simulink model "motominiPlanning"  (R2019a)
settings: Solver=ode3  StartTime=0.0  StopTime=totalTime  FixedStep=1e-3  RelTol=1e-3
values from neighbouring files (symbols this model uses):
  MotominiParams = setMotominiParameters(ROS_master_ip,motomini)    [managePlannerRequests.m]
  obstacles = [colObject1]    [calcStartingTrajWithPlanner.m]    (also in managePlannerRequests.m = []; testTrajectoryPlanner.m = [])
  Qt = QOpt    [calcStartingTrajWithPlanner.m]    (also in planTrajectory.m; testTrajectoryPlanner.m)
  s = char(axisElement.getAttribute('xyz'))    [loadRobotFromURDF.m]    (also in testTrajectoryPlanner.m = patch(surf2patch(X,Y,Z)))
  X = X + cupPosition(1)    [testTrajectoryPlanner.m]
  Y = Y + cupPosition(2)    [testTrajectoryPlanner.m]
  Z = Z + cupPosition(3)    [testTrajectoryPlanner.m]
undefined symbols (not defined in the file or in its folder): X0, Xf
libraries: sm_lib x111, nesl_utility x70, sharedtransform x2, aerolibtransform2 x2, simulink x1
(part 1 of 4)
settings Model: Creator=tomvose  LastModifiedBy=tkikawad
settings DataIOCC: ReturnWorkspaceOutputs=off
settings DebuggingCC: PregeneratedLibrarySubsystemCodeDiagnostic=none  ArithmeticOperatorsInVariantConditions=warning
settings SFSimCC: SimUseLocalCustomCode=off
settings RTWCC: RTWUseLocalCustomCode=off
settings CodeAppCC: StateflowObjectComments=on
settings ConfigComp: CovMetricSettings=dswe
settings SimscapeCC: SimscapeNormalizeSystem=off
settings ExplorerConfigSet: SimMechanicsOpenEditorOnUpdate=off

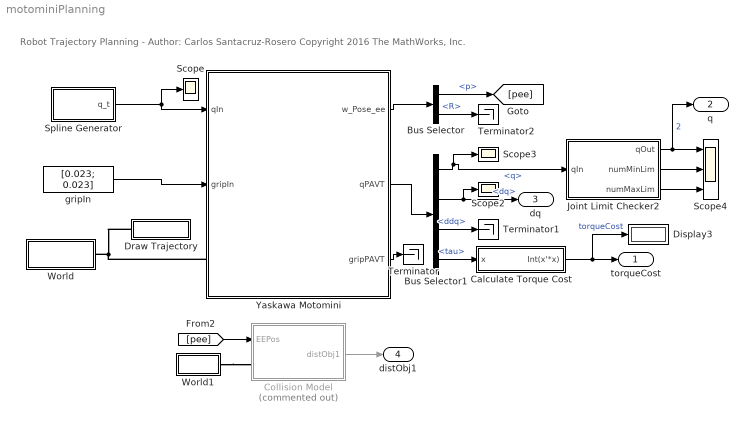
== system motominiPlanning ==
  note: Robot Trajectory Planning - Author: Carlos Santacruz-Rosero
      | Copyright 2016 The MathWorks, Inc.
  Bus Selector : BusSelector  OutputSignals=p,R
  Bus Selector1 : BusSelector  OutputSignals=q,dq,ddq,tau
  Calculate Torque Cost : Subsystem
  Collision Model : Subsystem  Commented=on
  Display3 : Display
  Draw Trajectory : Subsystem
  Joint Limit Checker2 : Subsystem  VariantControl="mode == OP2Model ||  mode == OP2ROS"
      mask Display:
      | plot([0.3 0.7], [0.5 0.5])
      | plot([0.3 0.4 0.6 0.7], [0.25 0.25 0.75 0.75])
  Scope : Scope
  Scope2 : Scope
  Scope3 : Scope
  Scope4 : Scope  NumInputPorts=3
  Spline Generator : Subsystem
  Terminator : Terminator
  Terminator1 : Terminator
  Terminator2 : Terminator
  World : Subsystem
  World1 : Subsystem
  Yaskawa Motomini : Subsystem
  gripIn : Constant  Value=[0.023; 0.023]
  torqueCost : Outport  SignalName=torqueCost
  q : Outport  Port=2  SignalName=q
  dq : Outport  Port=3  SignalName=dq
  distObj1 : Outport  Port=4  SignalName=distObj1
  wires:
  Spline Generator/1(q_t) -> Yaskawa Motomini/1(qIn), Scope/1
  gripIn/1 -> Yaskawa Motomini/2(gripIn)
  Yaskawa Motomini/1(w_Pose_ee) -> Bus Selector/1
  Yaskawa Motomini/2(qPAVT) -> Bus Selector1/1
  Yaskawa Motomini/3(gripPAVT) -> Terminator/1
  Bus Selector/1 -> [pee]  "<p>"
  Bus Selector/2 -> Terminator2/1  "<R>"
  Bus Selector1/1 -> Joint Limit Checker2/1(qIn), Scope3/1  "<q>"
  Bus Selector1/4 -> Calculate Torque Cost/1(x)  "<tau>"
  Calculate Torque Cost/1(Int(x'*x)) -> Display3/1, torqueCost/1  "torqueCost"
  [pee] -> Collision Model/1(EEPos)
  Collision Model/1(distObj1) -> distObj1/1
  Bus Selector1/2 -> Scope2/1, dq/1  "<dq>"
  Bus Selector1/3 -> Terminator1/1  "<ddq>"
  Joint Limit Checker2/2(numMinLim) -> Scope4/2
  Joint Limit Checker2/3(numMaxLim) -> Scope4/3
  Joint Limit Checker2/1(qOut) -> Scope4/1, q/1  "2"
  connections:
  Yaskawa Motomini/LConn1 -- Draw Trajectory/LConn1 -- World/RConn1
  World1/RConn1 -- Collision Model/LConn1

== system motominiPlanning/Calculate Torque Cost ==
  x : Inport
  Dot Product : DotProduct  InputSameDT=on  OutDataTypeStr=Inherit: Inherit via internal rule
  Integrator : Integrator
  Math Function : Math  Operator=transpose  SaturateOnIntegerOverflow=on
  Int(x'*x) : Outport
  wires:
  Dot Product/1 -> Integrator/1
  Math Function/1 -> Dot Product/1
  x/1 -> Dot Product/2, Math Function/1
  Integrator/1 -> Int(x'*x)/1

== system motominiPlanning/Collision Model ==
  EEPos : Inport
  Constant2 : Constant  Value=obstacles(1).pos
  Scope5 : Scope
  Sphere Collision Model : Subsystem
  Sphere Collision Object 1 : Subsystem  mask{R=0.05}
      mask prompts: R "Radius Sphere [m]"
  Sphere Collision Object 2 : Subsystem  mask{R=obstacles(1).radius}
      mask prompts: R "Radius Sphere [m]"
  c_base : PMIOPort  Side=Left
  distObj1 : Outport
  wires:
  Constant2/1 -> Sphere Collision Object 2/1(pos)
  Sphere Collision Object 1/1(sphereCO1) -> Sphere Collision Model/1(sphereCO1)
  Sphere Collision Object 2/1(sphereCO1) -> Sphere Collision Model/2(sphereCO2)
  Sphere Collision Model/2(hasCollision) -> Scope5/1
  Sphere Collision Model/1(distance) -> distObj1/1
  EEPos/1 -> Sphere Collision Object 1/1(pos)
  connections:
  Sphere Collision Object 1/LConn1 -- c_base/RConn1 -- Sphere Collision Object 2/LConn1

== system motominiPlanning/Draw Trajectory ==
  Draw Goal Task : Subsystem  mask{TaskPos=Xf.p, TaskEzyx=Xf.ezyx}
      mask prompts: TaskPos "Task Position"; TaskEzyx "Task Orientation (Exyz)"
  Draw Initial Task : Subsystem  Commented=on  mask{TaskPos=X0.p, TaskEzyx=X0.ezyx}
      mask prompts: TaskPos "Task Position"; TaskEzyx "Task Orientation (Exyz)"
  Optimal : sm_lib/Curves and Surfaces/Spline  DataPoints=XYZOpt  DataPointsUnits=m  EndConditionType=Natural  GraphicType=FromGeometry  MarkerShape=Sphere  MarkerSize=10  GraphicVisPropType=SimpleVisualProperties  GraphicDiffuseColor=[0.0 1.0 0.0]  GraphicSpecularColor=[0.5 0.5 0.5 1.0]  GraphicAmbientColor=[0.15 0.15 0.15 1.0]  GraphicEmissiveColor=[0.0 0.0 0.0 1.0]  GraphicShininess=75  GraphicOpacity=1.0
      settings: SourceProductName=Simscape Multibody
  Original : sm_lib/Curves and Surfaces/Spline  DataPoints=XYZOr  DataPointsUnits=m  EndConditionType=Natural  GraphicType=FromGeometry  MarkerShape=Sphere  MarkerSize=10  GraphicVisPropType=SimpleVisualProperties  GraphicDiffuseColor=[1.0 0.0 0.4]  GraphicSpecularColor=[0.5 0.5 0.5 1.0]  GraphicAmbientColor=[0.15 0.15 0.15 1.0]  GraphicEmissiveColor=[0.0 0.0 0.0 1.0]  GraphicShininess=75  GraphicOpacity=1.0
      settings: SourceProductName=Simscape Multibody
  c_base : PMIOPort  Side=Left
  connections:
  Draw Goal Task/LConn1 -- Original/LConn1 -- c_base/RConn1 -- Optimal/LConn1 -- Draw Initial Task/LConn1

== system motominiPlanning/Joint Limit Checker2 ==
  qIn : Inport
  Joint Limit Checker : MATLAB Function  TreatAsAtomicUnit=on  mask{qMin=MotominiParams.jntMinLim, qMax=MotominiParams.jntMaxLim}
      mask prompts: qMin "Min Joint Limits"; qMax "Max Joint Limits"
  qOut : Outport
  numMinLim : Outport  Port=2
  numMaxLim : Outport  Port=3
  wires:
  Joint Limit Checker/1(qOut) -> qOut/1
  qIn/1 -> Joint Limit Checker/1(qIn)
  Joint Limit Checker/3(numMaxLim) -> numMaxLim/1  "numMaxLim"
  Joint Limit Checker/2(numMinLim) -> numMinLim/1  "numMinLim"

== system motominiPlanning/Spline Generator ==
  note: Spline Generator
  1-D Lookup Table : Lookup_n-D  NumberOfTableDimensions=1  LookupTableObject=''  BreakpointsForDimension1=t  Table=Qt(1,:)  InterpMethod=Cubic spline  ExtrapMethod=Cubic spline  InternalRulePriority=Speed  RndMeth=Simplest  InputSameDT=on
  1-D Lookup Table1 : Lookup_n-D  NumberOfTableDimensions=1  LookupTableObject=''  BreakpointsForDimension1=t  Table=Qt(2,:)  InterpMethod=Cubic spline  ExtrapMethod=Cubic spline  InternalRulePriority=Speed  RndMeth=Simplest  InputSameDT=on
  1-D Lookup Table2 : Lookup_n-D  NumberOfTableDimensions=1  LookupTableObject=''  BreakpointsForDimension1=t  Table=Qt(3,:)  InterpMethod=Cubic spline  ExtrapMethod=Cubic spline  InternalRulePriority=Speed  RndMeth=Simplest  InputSameDT=on
  1-D Lookup Table3 : Lookup_n-D  NumberOfTableDimensions=1  LookupTableObject=''  BreakpointsForDimension1=t  Table=Qt(4,:)  InterpMethod=Cubic spline  ExtrapMethod=Cubic spline  InternalRulePriority=Speed  RndMeth=Simplest  InputSameDT=on
  1-D Lookup Table4 : Lookup_n-D  NumberOfTableDimensions=1  LookupTableObject=''  BreakpointsForDimension1=t  Table=Qt(5,:)  InterpMethod=Cubic spline  ExtrapMethod=Cubic spline  InternalRulePriority=Speed  RndMeth=Simplest  InputSameDT=on
  1-D Lookup Table5 : Lookup_n-D  NumberOfTableDimensions=1  LookupTableObject=''  BreakpointsForDimension1=t  Table=Qt(6,:)  InterpMethod=Cubic spline  ExtrapMethod=Cubic spline  InternalRulePriority=Speed  RndMeth=Simplest  InputSameDT=on
  Clock : Clock
  Mux : Mux  Inputs=6
  q_t : Outport
  wires:
  1-D Lookup Table2/1 -> Mux/3
  Clock/1 -> 1-D Lookup Table5/1, 1-D Lookup Table4/1, 1-D Lookup Table3/1, 1-D Lookup Table/1, 1-D Lookup Table1/1, 1-D Lookup Table2/1
  1-D Lookup Table4/1 -> Mux/5
  1-D Lookup Table3/1 -> Mux/4
  1-D Lookup Table/1 -> Mux/1
  Mux/1 -> q_t/1
  1-D Lookup Table1/1 -> Mux/2
  1-D Lookup Table5/1 -> Mux/6

== system motominiPlanning/World ==
  Mechanism Configuration : sm_lib/Utilities/Mechanism Configuration  UniformGravity=Constant  GravityVector=[0 0 -9.80665]  GravityUnits=m/s^2  LinearizationDelta=0.001
  Solver Configuration : nesl_utility/Solver Configuration  PhysicalDomain=network_engine_domain  SubClassName=solver  LeftPortType=input  RightPortType=generic  Tones=[]  Harmonics=[]  SimulateNoise=off  Profile=off  UseLocalSampling=off  EnableSwitchedLinearOptims=on  FrequencyDomain=off  UseCCode=off  RelTol=0.001  AbsTol=1e-06  MinStep=1e-09  ToWorkspace=off  RevertToSquareIcSolve=off  NumHomotopyIterations=100  PhasorMode=off  PhasorModeNumHarmonics=1  DoDC=off  ResidualTolerance=1e-09  UseLocalSolver=off  LocalSolverChoice=NE_BACKWARD_EULER_ADVANCER  LocalSolverSampleTime=0.001  DoFixedCost=off  MaxNonlinIter=3  MaxModeIter=2  LinearAlgebra=Sparse  EquationFormulation=NE_TIME_EF  DelaysMemoryBudget=1024  AutomaticFiltering=on  FilteringTimeConstant=0.001  PartitionStorageMethod=AS_NEEDED  PartitionMemoryBudget=1024  PartitionMethod=FAST
  World Frame : sm_lib/Frames and Transforms/World Frame
  c_world : PMIOPort  Side=Right
  connections:
  Mechanism Configuration/RConn1 -- c_world/RConn1 -- Solver Configuration/RConn1 -- World Frame/RConn1

== system motominiPlanning/World1 ==
  Mechanism Configuration : sm_lib/Utilities/Mechanism Configuration  UniformGravity=Constant  GravityVector=[0 0 -9.80665]  GravityUnits=m/s^2  LinearizationDelta=0.001
  Solver Configuration : nesl_utility/Solver Configuration  PhysicalDomain=network_engine_domain  SubClassName=solver  LeftPortType=input  RightPortType=generic  Tones=[]  Harmonics=[]  SimulateNoise=off  Profile=off  UseLocalSampling=off  EnableSwitchedLinearOptims=on  FrequencyDomain=off  UseCCode=off  RelTol=0.001  AbsTol=1e-06  MinStep=1e-09  ToWorkspace=off  RevertToSquareIcSolve=off  NumHomotopyIterations=100  PhasorMode=off  PhasorModeNumHarmonics=1  DoDC=off  ResidualTolerance=1e-09  UseLocalSolver=off  LocalSolverChoice=NE_BACKWARD_EULER_ADVANCER  LocalSolverSampleTime=0.001  DoFixedCost=off  MaxNonlinIter=3  MaxModeIter=2  LinearAlgebra=Sparse  EquationFormulation=NE_TIME_EF  DelaysMemoryBudget=1024  AutomaticFiltering=on  FilteringTimeConstant=0.001  PartitionStorageMethod=AS_NEEDED  PartitionMemoryBudget=1024  PartitionMethod=FAST
  World Frame : sm_lib/Frames and Transforms/World Frame
  c_world : PMIOPort  Side=Right
  connections:
  World Frame/RConn1 -- Solver Configuration/RConn1 -- c_world/RConn1 -- Mechanism Configuration/RConn1

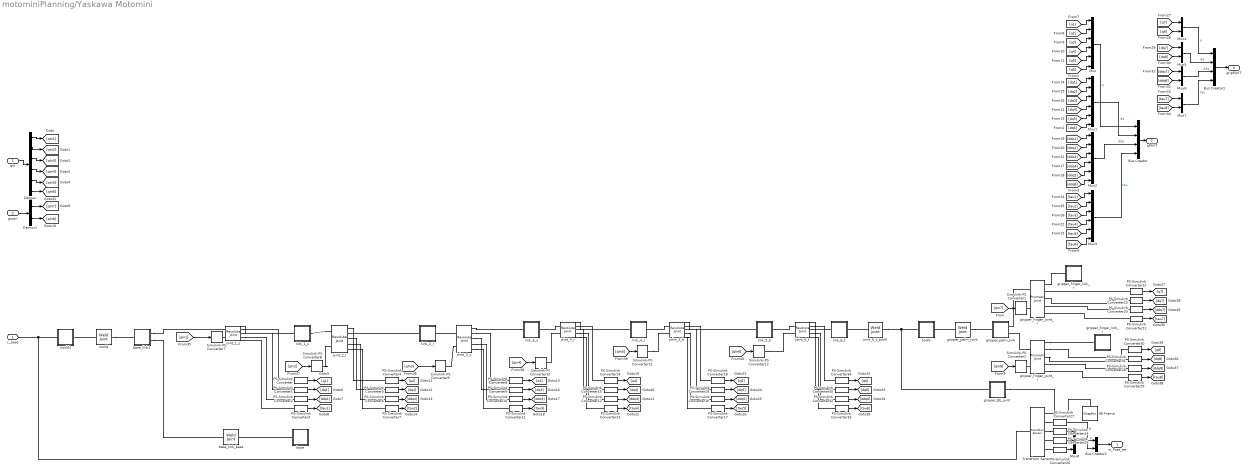
== system motominiPlanning/Yaskawa Motomini ==
  qIn : Inport
  gripIn : Inport  Port=2
  Bus Creator : BusCreator  Inputs=4
  Bus Creator1 : BusCreator  Inputs=4
  Bus Creator2 : BusCreator  Inputs=2
  Demux : Demux  Outputs=6
  Demux1 : Demux  Outputs=2
  EE Frame : sm_lib/Body Elements/Graphic  GraphicType=Marker  MarkerShape=Frame  MarkerSize=40  GraphicVisPropType=SimpleVisualProperties  GraphicDiffuseColor=[1.0 0.6 0.0]  GraphicSpecularColor=[0.5 0.5 0.5 1.0]  GraphicAmbientColor=[0.15 0.15 0.15 1.0]  GraphicEmissiveColor=[0.0 0.0 0.0 1.0]  GraphicShininess=75  GraphicOpacity=1.0
      settings: SourceProductName=Simscape Multibody
  Mux{,1..3} (4 alike) : Mux  Inputs=6
  Mux{4..7} (4 alike) : Mux  Inputs=2
  Mux8 : Mux  Inputs=3
  PS-Simulink Converter{,1..35} (36 alike) : nesl_utility/PS-Simulink Converter  PhysicalDomain=network_engine_domain  SubClassName=ps_output  LeftPortType=input  RightPortType=output  PseudoPeriodic=off  Frequencies=[]  Unit=1  AffineConversion=off
  Simulink-PS Converter{1..2,11..12} (4 alike) : nesl_utility/Simulink-PS Converter  PhysicalDomain=network_engine_domain  SubClassName=ps_input  LeftPortType=input  RightPortType=output  PseudoPeriodic=off  Frequencies=[]  NoiseDistribution=none  NoiseParameters=[]  Unit=1  AffineConversion=off  FilteringAndDerivatives=filter  SimscapeFilterOrder=2  InputFilterTimeConstant=0.001  UdotUserProvided=2
  Simulink-PS Converter{7..10} (4 alike) : nesl_utility/Simulink-PS Converter  PhysicalDomain=network_engine_domain  SubClassName=ps_input  LeftPortType=input  RightPortType=output  PseudoPeriodic=off  Frequencies=[]  NoiseDistribution=none  NoiseParameters=[]  Unit=1  AffineConversion=off  FilteringAndDerivatives=filter  SimscapeFilterOrder=2  InputFilterTimeConstant=0.001  UdotUserProvided=1
  Transform Sensor : sm_lib/Frames and Transforms/Transform Sensor  MeasurementFrame=World  SenseAngle=off  SenseAxis=off  SenseAngle1=off  SenseAngle2=off  SenseAngle3=off  SenseQ=off  SenseR=on  SenseOmegaX=off  SenseOmegaY=off  SenseOmegaZ=off  SenseOmega1=off  SenseOmega2=off  SenseOmega3=off  SenseQDot=off  SenseRDot=off  SenseAlphaX=off  SenseAlphaY=off  SenseAlphaZ=off  SenseAlpha1=off  SenseAlpha2=off  SenseAlpha3=off  SenseQDDot=off  SenseRDDot=off  SenseX=on  SenseY=on  SenseZ=on  SenseRad=off  SenseAzim=off  SenseDist=off  SenseInc=off  SenseXDot=off  SenseYDot=off  SenseZDot=off  SenseRadDot=off  SenseAzimDot=off  SenseDistDot=off  SenseIncDot=off  SenseXDDot=off  SenseYDDot=off  SenseZDDot=off  SenseRadDDot=off  SenseAzimDDot=off  SenseDistDDot=off  SenseIncDDot=off
  base : Subsystem
  base_link1 : Subsystem
  base_link_base : sm_lib/Joints/Weld Joint  SenseConstraintForce=off  SenseConstraintForceX=off  SenseConstraintForceY=off  SenseConstraintForceZ=off  SenseConstraintTorque=off  SenseConstraintTorqueX=off  SenseConstraintTorqueY=off  SenseConstraintTorqueZ=off  SenseTotalForce=off  SenseTotalForceX=off  SenseTotalForceY=off  SenseTotalForceZ=off  SenseTotalTorque=off  SenseTotalTorqueX=off  SenseTotalTorqueY=off  SenseTotalTorqueZ=off  CompositeWrenchDir=FollowerOnBase  CompositeWrenchFrame=BaseFrame
  gripper_EE_joint : Subsystem
  gripper_finger_joint_l : sm_lib/Joints/Prismatic Joint  SenseConstraintForce=off  SenseConstraintForceX=off  SenseConstraintForceY=off  SenseConstraintForceZ=off  SenseConstraintTorque=off  SenseConstraintTorqueX=off  SenseConstraintTorqueY=off  SenseConstraintTorqueZ=off  SenseTotalForce=off  SenseTotalForceX=off  SenseTotalForceY=off  SenseTotalForceZ=off  SenseTotalTorque=off  SenseTotalTorqueX=off  SenseTotalTorqueY=off  SenseTotalTorqueZ=off  CompositeWrenchDir=FollowerOnBase  CompositeWrenchFrame=BaseFrame  EquilibriumPosition=0  EquilibriumPositionUnits=m  SpringStiffness=0  SpringStiffnessUnits=N/m  DampingCoefficient=1  DampingCoefficientUnits=kg/s  TorqueActuationMode=ComputedTorque  MotionActuationMode=InputMotion  SensePosition=on  SenseVelocity=on  SenseAcceleration=on  SenseTorqueForce=on  SenseLowerLimitTorqueForce=off  SenseUpperLimitTorqueForce=off  LowerLimitSpecify=off  LowerLimitBound=-1  LowerLimitBoundUnits=m  LowerLimitStiffness=1e6  LowerLimitStiffnessUnits=N/m  LowerLimitDamping=1e3  LowerLimitDampingUnits=N/(m/s)  LowerLimitTransitionRegionWidth=1e-4  LowerLimitTransitionRegionWidthUnits=m  UpperLimitSpecify=off  UpperLimitBound=1  UpperLimitBoundUnits=m  UpperLimitStiffness=1e6  UpperLimitStiffnessUnits=N/m  UpperLimitDamping=1e3  UpperLimitDampingUnits=N/(m/s)  UpperLimitTransitionRegionWidth=1e-4  UpperLimitTransitionRegionWidthUnits=m  PositionTargetSpecify=off  PositionTargetPriority=High  PositionTargetValue=0  PositionTargetValueUnits=m  VelocityTargetSpecify=off  VelocityTargetPriority=High  VelocityTargetValue=0  VelocityTargetValueUnits=m/s
  gripper_finger_joint_r : sm_lib/Joints/Prismatic Joint  SenseConstraintForce=off  SenseConstraintForceX=off  SenseConstraintForceY=off  SenseConstraintForceZ=off  SenseConstraintTorque=off  SenseConstraintTorqueX=off  SenseConstraintTorqueY=off  SenseConstraintTorqueZ=off  SenseTotalForce=off  SenseTotalForceX=off  SenseTotalForceY=off  SenseTotalForceZ=off  SenseTotalTorque=off  SenseTotalTorqueX=off  SenseTotalTorqueY=off  SenseTotalTorqueZ=off  CompositeWrenchDir=FollowerOnBase  CompositeWrenchFrame=BaseFrame  EquilibriumPosition=0  EquilibriumPositionUnits=m  SpringStiffness=0  SpringStiffnessUnits=N/m  DampingCoefficient=1  DampingCoefficientUnits=kg/s  TorqueActuationMode=ComputedTorque  MotionActuationMode=InputMotion  SensePosition=on  SenseVelocity=on  SenseAcceleration=on  SenseTorqueForce=on  SenseLowerLimitTorqueForce=off  SenseUpperLimitTorqueForce=off  LowerLimitSpecify=off  LowerLimitBound=-1  LowerLimitBoundUnits=m  LowerLimitStiffness=1e6  LowerLimitStiffnessUnits=N/m  LowerLimitDamping=1e3  LowerLimitDampingUnits=N/(m/s)  LowerLimitTransitionRegionWidth=1e-4  LowerLimitTransitionRegionWidthUnits=m  UpperLimitSpecify=off  UpperLimitBound=1  UpperLimitBoundUnits=m  UpperLimitStiffness=1e6  UpperLimitStiffnessUnits=N/m  UpperLimitDamping=1e3  UpperLimitDampingUnits=N/(m/s)  UpperLimitTransitionRegionWidth=1e-4  UpperLimitTransitionRegionWidthUnits=m  PositionTargetSpecify=off  PositionTargetPriority=High  PositionTargetValue=0  PositionTargetValueUnits=m  VelocityTargetSpecify=off  VelocityTargetPriority=High  VelocityTargetValue=0  VelocityTargetValueUnits=m/s
  gripper_finger_link_l : Subsystem
  gripper_finger_link_r : Subsystem
  gripper_palm_joint : sm_lib/Joints/Weld Joint  SenseConstraintForce=off  SenseConstraintForceX=off  SenseConstraintForceY=off  SenseConstraintForceZ=off  SenseConstraintTorque=off  SenseConstraintTorqueX=off  SenseConstraintTorqueY=off  SenseConstraintTorqueZ=off  SenseTotalForce=off  SenseTotalForceX=off  SenseTotalForceY=off  SenseTotalForceZ=off  SenseTotalTorque=off  SenseTotalTorqueX=off  SenseTotalTorqueY=off  SenseTotalTorqueZ=off  CompositeWrenchDir=FollowerOnBase  CompositeWrenchFrame=BaseFrame
  gripper_palm_link : Subsystem
  joint_1_s : sm_lib/Joints/Revolute Joint  SenseConstraintForce=off  SenseConstraintForceX=off  SenseConstraintForceY=off  SenseConstraintForceZ=off  SenseConstraintTorque=off  SenseConstraintTorqueX=off  SenseConstraintTorqueY=off  SenseConstraintTorqueZ=off  SenseTotalForce=off  SenseTotalForceX=off  SenseTotalForceY=off  SenseTotalForceZ=off  SenseTotalTorque=off  SenseTotalTorqueX=off  SenseTotalTorqueY=off  SenseTotalTorqueZ=off  CompositeWrenchDir=FollowerOnBase  CompositeWrenchFrame=BaseFrame  EquilibriumPosition=0  EquilibriumPositionUnits=deg  SpringStiffness=0  SpringStiffnessUnits=N*m/deg  DampingCoefficient=0  DampingCoefficientUnits=m^2*kg/s/rad  TorqueActuationMode=ComputedTorque  MotionActuationMode=InputMotion  SensePosition=on  SenseVelocity=on  SenseAcceleration=on  SenseTorqueForce=on  SenseLowerLimitTorqueForce=off  SenseUpperLimitTorqueForce=off  LowerLimitSpecify=off  LowerLimitBound=-90  LowerLimitBoundUnits=deg  LowerLimitStiffness=1e4  LowerLimitStiffnessUnits=N*m/deg  LowerLimitDamping=10  LowerLimitDampingUnits=N*m/(deg/s)  LowerLimitTransitionRegionWidth=0.1  LowerLimitTransitionRegionWidthUnits=deg  UpperLimitSpecify=off  UpperLimitBound=90  UpperLimitBoundUnits=deg  UpperLimitStiffness=1e4  UpperLimitStiffnessUnits=N*m/deg  UpperLimitDamping=10  UpperLimitDampingUnits=N*m/(deg/s)  UpperLimitTransitionRegionWidth=0.1  UpperLimitTransitionRegionWidthUnits=deg  PositionTargetSpecify=on  PositionTargetPriority=High  PositionTargetValue=0  PositionTargetValueUnits=deg  VelocityTargetSpecify=off  VelocityTargetPriority=High  VelocityTargetValue=0  VelocityTargetValueUnits=deg/s
  joint_2_l : sm_lib/Joints/Revolute Joint  SenseConstraintForce=off  SenseConstraintForceX=off  SenseConstraintForceY=off  SenseConstraintForceZ=off  SenseConstraintTorque=off  SenseConstraintTorqueX=off  SenseConstraintTorqueY=off  SenseConstraintTorqueZ=off  SenseTotalForce=off  SenseTotalForceX=off  SenseTotalForceY=off  SenseTotalForceZ=off  SenseTotalTorque=off  SenseTotalTorqueX=off  SenseTotalTorqueY=off  SenseTotalTorqueZ=off  CompositeWrenchDir=FollowerOnBase  CompositeWrenchFrame=BaseFrame  EquilibriumPosition=0  EquilibriumPositionUnits=deg  SpringStiffness=0  SpringStiffnessUnits=N*m/deg  DampingCoefficient=0  DampingCoefficientUnits=m^2*kg/s/rad  TorqueActuationMode=ComputedTorque  MotionActuationMode=InputMotion  SensePosition=on  SenseVelocity=on  SenseAcceleration=on  SenseTorqueForce=on  SenseLowerLimitTorqueForce=off  SenseUpperLimitTorqueForce=off  LowerLimitSpecify=off  LowerLimitBound=-90  LowerLimitBoundUnits=deg  LowerLimitStiffness=1e4  LowerLimitStiffnessUnits=N*m/deg  LowerLimitDamping=10  LowerLimitDampingUnits=N*m/(deg/s)  LowerLimitTransitionRegionWidth=0.1  LowerLimitTransitionRegionWidthUnits=deg  UpperLimitSpecify=off  UpperLimitBound=90  UpperLimitBoundUnits=deg  UpperLimitStiffness=1e4  UpperLimitStiffnessUnits=N*m/deg  UpperLimitDamping=10  UpperLimitDampingUnits=N*m/(deg/s)  UpperLimitTransitionRegionWidth=0.1  UpperLimitTransitionRegionWidthUnits=deg  PositionTargetSpecify=on  PositionTargetPriority=High  PositionTargetValue=0  PositionTargetValueUnits=deg  VelocityTargetSpecify=off  VelocityTargetPriority=High  VelocityTargetValue=0  VelocityTargetValueUnits=deg/s
  joint_3_u : sm_lib/Joints/Revolute Joint  SenseConstraintForce=off  SenseConstraintForceX=off  SenseConstraintForceY=off  SenseConstraintForceZ=off  SenseConstraintTorque=off  SenseConstraintTorqueX=off  SenseConstraintTorqueY=off  SenseConstraintTorqueZ=off  SenseTotalForce=off  SenseTotalForceX=off  SenseTotalForceY=off  SenseTotalForceZ=off  SenseTotalTorque=off  SenseTotalTorqueX=off  SenseTotalTorqueY=off  SenseTotalTorqueZ=off  CompositeWrenchDir=FollowerOnBase  CompositeWrenchFrame=BaseFrame  EquilibriumPosition=0  EquilibriumPositionUnits=deg  SpringStiffness=0  SpringStiffnessUnits=N*m/deg  DampingCoefficient=0  DampingCoefficientUnits=m^2*kg/s/rad  TorqueActuationMode=ComputedTorque  MotionActuationMode=InputMotion  SensePosition=on  SenseVelocity=on  SenseAcceleration=on  SenseTorqueForce=on  SenseLowerLimitTorqueForce=off  SenseUpperLimitTorqueForce=off  LowerLimitSpecify=off  LowerLimitBound=-90  LowerLimitBoundUnits=deg  LowerLimitStiffness=1e4  LowerLimitStiffnessUnits=N*m/deg  LowerLimitDamping=10  LowerLimitDampingUnits=N*m/(deg/s)  LowerLimitTransitionRegionWidth=0.1  LowerLimitTransitionRegionWidthUnits=deg  UpperLimitSpecify=off  UpperLimitBound=90  UpperLimitBoundUnits=deg  UpperLimitStiffness=1e4  UpperLimitStiffnessUnits=N*m/deg  UpperLimitDamping=10  UpperLimitDampingUnits=N*m/(deg/s)  UpperLimitTransitionRegionWidth=0.1  UpperLimitTransitionRegionWidthUnits=deg  PositionTargetSpecify=on  PositionTargetPriority=High  PositionTargetValue=0  PositionTargetValueUnits=deg  VelocityTargetSpecify=off  VelocityTargetPriority=High  VelocityTargetValue=0  VelocityTargetValueUnits=deg/s
  joint_4_r : sm_lib/Joints/Revolute Joint  SenseConstraintForce=off  SenseConstraintForceX=off  SenseConstraintForceY=off  SenseConstraintForceZ=off  SenseConstraintTorque=off  SenseConstraintTorqueX=off  SenseConstraintTorqueY=off  SenseConstraintTorqueZ=off  SenseTotalForce=off  SenseTotalForceX=off  SenseTotalForceY=off  SenseTotalForceZ=off  SenseTotalTorque=off  SenseTotalTorqueX=off  SenseTotalTorqueY=off  SenseTotalTorqueZ=off  CompositeWrenchDir=FollowerOnBase  CompositeWrenchFrame=BaseFrame  EquilibriumPosition=0  EquilibriumPositionUnits=deg  SpringStiffness=0  SpringStiffnessUnits=N*m/deg  DampingCoefficient=0  DampingCoefficientUnits=m^2*kg/s/rad  TorqueActuationMode=ComputedTorque  MotionActuationMode=InputMotion  SensePosition=on  SenseVelocity=on  SenseAcceleration=on  SenseTorqueForce=on  SenseLowerLimitTorqueForce=off  SenseUpperLimitTorqueForce=off  LowerLimitSpecify=off  LowerLimitBound=-90  LowerLimitBoundUnits=deg  LowerLimitStiffness=1e4  LowerLimitStiffnessUnits=N*m/deg  LowerLimitDamping=10  LowerLimitDampingUnits=N*m/(deg/s)  LowerLimitTransitionRegionWidth=0.1  LowerLimitTransitionRegionWidthUnits=deg  UpperLimitSpecify=off  UpperLimitBound=90  UpperLimitBoundUnits=deg  UpperLimitStiffness=1e4  UpperLimitStiffnessUnits=N*m/deg  UpperLimitDamping=10  UpperLimitDampingUnits=N*m/(deg/s)  UpperLimitTransitionRegionWidth=0.1  UpperLimitTransitionRegionWidthUnits=deg  PositionTargetSpecify=on  PositionTargetPriority=High  PositionTargetValue=0  PositionTargetValueUnits=deg  VelocityTargetSpecify=off  VelocityTargetPriority=High  VelocityTargetValue=0  VelocityTargetValueUnits=deg/s
  joint_5_b : sm_lib/Joints/Revolute Joint  SenseConstraintForce=off  SenseConstraintForceX=off  SenseConstraintForceY=off  SenseConstraintForceZ=off  SenseConstraintTorque=off  SenseConstraintTorqueX=off  SenseConstraintTorqueY=off  SenseConstraintTorqueZ=off  SenseTotalForce=off  SenseTotalForceX=off  SenseTotalForceY=off  SenseTotalForceZ=off  SenseTotalTorque=off  SenseTotalTorqueX=off  SenseTotalTorqueY=off  SenseTotalTorqueZ=off  CompositeWrenchDir=FollowerOnBase  CompositeWrenchFrame=BaseFrame  EquilibriumPosition=0  EquilibriumPositionUnits=deg  SpringStiffness=0  SpringStiffnessUnits=N*m/deg  DampingCoefficient=0  DampingCoefficientUnits=m^2*kg/s/rad  TorqueActuationMode=ComputedTorque  MotionActuationMode=InputMotion  SensePosition=on  SenseVelocity=on  SenseAcceleration=on  SenseTorqueForce=on  SenseLowerLimitTorqueForce=off  SenseUpperLimitTorqueForce=off  LowerLimitSpecify=off  LowerLimitBound=-90  LowerLimitBoundUnits=deg  LowerLimitStiffness=1e4  LowerLimitStiffnessUnits=N*m/deg  LowerLimitDamping=10  LowerLimitDampingUnits=N*m/(deg/s)  LowerLimitTransitionRegionWidth=0.1  LowerLimitTransitionRegionWidthUnits=deg  UpperLimitSpecify=off  UpperLimitBound=90  UpperLimitBoundUnits=deg  UpperLimitStiffness=1e4  UpperLimitStiffnessUnits=N*m/deg  UpperLimitDamping=10  UpperLimitDampingUnits=N*m/(deg/s)  UpperLimitTransitionRegionWidth=0.1  UpperLimitTransitionRegionWidthUnits=deg  PositionTargetSpecify=on  PositionTargetPriority=High  PositionTargetValue=0  PositionTargetValueUnits=deg  VelocityTargetSpecify=off  VelocityTargetPriority=High  VelocityTargetValue=0  VelocityTargetValueUnits=deg/s
  joint_6_t : sm_lib/Joints/Revolute Joint  SenseConstraintForce=off  SenseConstraintForceX=off  SenseConstraintForceY=off  SenseConstraintForceZ=off  SenseConstraintTorque=off  SenseConstraintTorqueX=off  SenseConstraintTorqueY=off  SenseConstraintTorqueZ=off  SenseTotalForce=off  SenseTotalForceX=off  SenseTotalForceY=off  SenseTotalForceZ=off  SenseTotalTorque=off  SenseTotalTorqueX=off  SenseTotalTorqueY=off  SenseTotalTorqueZ=off  CompositeWrenchDir=FollowerOnBase  CompositeWrenchFrame=BaseFrame  EquilibriumPosition=0  EquilibriumPositionUnits=deg  SpringStiffness=0  SpringStiffnessUnits=N*m/deg  DampingCoefficient=0  DampingCoefficientUnits=m^2*kg/s/rad  TorqueActuationMode=ComputedTorque  MotionActuationMode=InputMotion  SensePosition=on  SenseVelocity=on  SenseAcceleration=on  SenseTorqueForce=on  SenseLowerLimitTorqueForce=off  SenseUpperLimitTorqueForce=off  LowerLimitSpecify=off  LowerLimitBound=-90  LowerLimitBoundUnits=deg  LowerLimitStiffness=1e4  LowerLimitStiffnessUnits=N*m/deg  LowerLimitDamping=10  LowerLimitDampingUnits=N*m/(deg/s)  LowerLimitTransitionRegionWidth=0.1  LowerLimitTransitionRegionWidthUnits=deg  UpperLimitSpecify=off  UpperLimitBound=90  UpperLimitBoundUnits=deg  UpperLimitStiffness=1e4  UpperLimitStiffnessUnits=N*m/deg  UpperLimitDamping=10  UpperLimitDampingUnits=N*m/(deg/s)  UpperLimitTransitionRegionWidth=0.1  UpperLimitTransitionRegionWidthUnits=deg  PositionTargetSpecify=on  PositionTargetPriority=High  PositionTargetValue=0  PositionTargetValueUnits=deg  VelocityTargetSpecify=off  VelocityTargetPriority=High  VelocityTargetValue=0  VelocityTargetValueUnits=deg/s
  joint_6_t_tool0 : sm_lib/Joints/Weld Joint  SenseConstraintForce=off  SenseConstraintForceX=off  SenseConstraintForceY=off  SenseConstraintForceZ=off  SenseConstraintTorque=off  SenseConstraintTorqueX=off  SenseConstraintTorqueY=off  SenseConstraintTorqueZ=off  SenseTotalForce=off  SenseTotalForceX=off  SenseTotalForceY=off  SenseTotalForceZ=off  SenseTotalTorque=off  SenseTotalTorqueX=off  SenseTotalTorqueY=off  SenseTotalTorqueZ=off  CompositeWrenchDir=FollowerOnBase  CompositeWrenchFrame=BaseFrame
  link_1_s : Subsystem
  link_2_l : Subsystem
  link_3_u : Subsystem
  link_4_r : Subsystem
  link_5_b : Subsystem
  link_6_t : Subsystem
  tool0 : Subsystem
  world : sm_lib/Joints/Weld Joint  SenseConstraintForce=off  SenseConstraintForceX=off  SenseConstraintForceY=off  SenseConstraintForceZ=off  SenseConstraintTorque=off  SenseConstraintTorqueX=off  SenseConstraintTorqueY=off  SenseConstraintTorqueZ=off  SenseTotalForce=off  SenseTotalForceX=off  SenseTotalForceY=off  SenseTotalForceZ=off  SenseTotalTorque=off  SenseTotalTorqueX=off  SenseTotalTorqueY=off  SenseTotalTorqueZ=off  CompositeWrenchDir=FollowerOnBase  CompositeWrenchFrame=BaseFrame
  world1 : Subsystem
  c_base : PMIOPort  Side=Left
  w_Pose_ee : Outport
  qPAVT : Outport  Port=2
  gripPAVT : Outport  Port=3
  wires:
  Demux/1 -> [qIn1]
  Demux/2 -> [qIn2]
  Demux/3 -> [qIn3]
  Demux/4 -> [qIn4]
  Demux/5 -> [qIn5]
  qIn/1 -> Demux/1
  Demux1/1 -> [qIn7]
  Demux1/2 -> [qIn8]
  gripIn/1 -> Demux1/1
  [q1] -> Mux/1
  [q2] -> Mux/2
  [q3] -> Mux/3
  [q4] -> Mux/4
  [q5] -> Mux/5
  Mux/1 -> Bus Creator/1  "q"
  [dq1] -> Mux1/1
  [dq2] -> Mux1/2
  [dq3] -> Mux1/3
  [dq4] -> Mux1/4
  [dq5] -> Mux1/5
  Mux1/1 -> Bus Creator/2  "dq"
  [ddq1] -> Mux2/1
  [ddq2] -> Mux2/2
  [ddq3] -> Mux2/3
  [ddq4] -> Mux2/4
  [ddq5] -> Mux2/5
  Mux2/1 -> Bus Creator/3  "ddq"
  [tau1] -> Mux3/1
  [tau2] -> Mux3/2
  [tau3] -> Mux3/3
  [tau4] -> Mux3/4
  [tau5] -> Mux3/5
  Mux3/1 -> Bus Creator/4  "tau"
  [q7] -> Mux4/1
  [q8] -> Mux4/2
  [dq7] -> Mux5/1
  [dq8] -> Mux5/2
  [ddq7] -> Mux6/1
  [ddq8] -> Mux6/2
  [tau7] -> Mux7/1
  [tau8] -> Mux7/2
  Bus Creator/1 -> qPAVT/1
  Mux4/1 -> Bus Creator1/1  "q"
  Mux5/1 -> Bus Creator1/2  "dq"
  Mux6/1 -> Bus Creator1/3  "ddq"
  Mux7/1 -> Bus Creator1/4  "tau"
  Bus Creator1/1 -> gripPAVT/1
  PS-Simulink Converter24/1 -> Mux8/1
  PS-Simulink Converter25/1 -> Mux8/2
  PS-Simulink Converter26/1 -> Mux8/3
  Mux8/1 -> Bus Creator2/1  "p"
  PS-Simulink Converter27/1 -> Bus Creator2/2  "R"
  Bus Creator2/1 -> w_Pose_ee/1
  [qIn1] -> Simulink-PS Converter7/1
  [qIn2] -> Simulink-PS Converter8/1
  [qIn3] -> Simulink-PS Converter9/1
  [qIn4] -> Simulink-PS Converter10/1
  [qIn5] -> Simulink-PS Converter11/1
  [qIn6] -> Simulink-PS Converter12/1
  Demux/6 -> [qIn6]
  PS-Simulink Converter3/1 -> [tau1]
  PS-Simulink Converter1/1 -> [dq1]
  PS-Simulink Converter2/1 -> [ddq1]
  PS-Simulink Converter/1 -> [q1]
  PS-Simulink Converter7/1 -> [tau2]
  PS-Simulink Converter4/1 -> [q2]
  PS-Simulink Converter5/1 -> [dq2]
  PS-Simulink Converter6/1 -> [ddq2]
  PS-Simulink Converter9/1 -> [dq3]
  PS-Simulink Converter11/1 -> [tau3]
  PS-Simulink Converter8/1 -> [q3]
  PS-Simulink Converter10/1 -> [ddq3]
  PS-Simulink Converter13/1 -> [tau4]
  PS-Simulink Converter12/1 -> [ddq4]
  PS-Simulink Converter14/1 -> [q4]
  PS-Simulink Converter15/1 -> [dq4]
  PS-Simulink Converter19/1 -> [dq5]
  PS-Simulink Converter18/1 -> [q5]
  PS-Simulink Converter17/1 -> [tau5]
  PS-Simulink Converter16/1 -> [ddq5]
  PS-Simulink Converter32/1 -> [ddq6]
  PS-Simulink Converter33/1 -> [tau6]
  PS-Simulink Converter34/1 -> [q6]
  PS-Simulink Converter35/1 -> [dq6]
  [q6] -> Mux/6
  [dq6] -> Mux1/6
  [ddq6] -> Mux2/6
  [tau6] -> Mux3/6
  [qIn7] -> Simulink-PS Converter1/1
  [qIn8] -> Simulink-PS Converter2/1
  PS-Simulink Converter23/1 -> [dq7]
  PS-Simulink Converter22/1 -> [q7]
  PS-Simulink Converter21/1 -> [tau7]
  PS-Simulink Converter20/1 -> [ddq7]
  PS-Simulink Converter28/1 -> [ddq8]
  PS-Simulink Converter29/1 -> [tau8]
  PS-Simulink Converter30/1 -> [q8]
  PS-Simulink Converter31/1 -> [dq8]
  connections:
  Transform Sensor/RConn3 -- PS-Simulink Converter24/LConn1
  PS-Simulink Converter25/LConn1 -- Transform Sensor/RConn4
  PS-Simulink Converter26/LConn1 -- Transform Sensor/RConn5
  PS-Simulink Converter27/LConn1 -- Transform Sensor/RConn2
  base/LConn1 -- base_link_base/RConn1
  joint_6_t_tool0/LConn1 -- link_6_t/RConn1
  joint_1_s/RConn1 -- link_1_s/LConn1
  joint_2_l/LConn1 -- link_1_s/RConn1
  joint_4_r/LConn1 -- link_3_u/RConn1
  joint_6_t/RConn1 -- link_6_t/LConn1
  Transform Sensor/LConn1 -- world1/LConn1 -- c_base/RConn1
  joint_5_b/RConn1 -- link_5_b/LConn1
  joint_6_t_tool0/RConn1 -- gripper_EE_joint/LConn1 -- tool0/LConn1
  joint_2_l/RConn1 -- link_2_l/LConn1
  joint_3_u/LConn1 -- link_2_l/RConn1
  joint_3_u/RConn1 -- link_3_u/LConn1
  base_link1/RConn1 -- joint_1_s/LConn1
  joint_5_b/LConn1 -- link_4_r/RConn1
  base_link1/RConn2 -- base_link_base/LConn1
  joint_6_t/LConn1 -- link_5_b/RConn1
  joint_4_r/RConn1 -- link_4_r/LConn1
  joint_1_s/LConn2 -- Simulink-PS Converter7/RConn1
  Simulink-PS Converter8/RConn1 -- joint_2_l/LConn2
  Simulink-PS Converter9/RConn1 -- joint_3_u/LConn2
  Simulink-PS Converter10/RConn1 -- joint_4_r/LConn2
  Simulink-PS Converter11/RConn1 -- joint_5_b/LConn2
  Simulink-PS Converter12/RConn1 -- joint_6_t/LConn2
  joint_1_s/RConn3 -- PS-Simulink Converter1/LConn1
  joint_1_s/RConn4 -- PS-Simulink Converter2/LConn1
  PS-Simulink Converter/LConn1 -- joint_1_s/RConn2
  PS-Simulink Converter3/LConn1 -- joint_1_s/RConn5
  joint_2_l/RConn4 -- PS-Simulink Converter6/LConn1
  joint_2_l/RConn5 -- PS-Simulink Converter7/LConn1
  joint_2_l/RConn2 -- PS-Simulink Converter4/LConn1
  joint_2_l/RConn3 -- PS-Simulink Converter5/LConn1
  joint_3_u/RConn3 -- PS-Simulink Converter9/LConn1
  joint_3_u/RConn4 -- PS-Simulink Converter10/LConn1
  joint_3_u/RConn2 -- PS-Simulink Converter8/LConn1
  joint_3_u/RConn5 -- PS-Simulink Converter11/LConn1
  joint_4_r/RConn5 -- PS-Simulink Converter13/LConn1
  joint_4_r/RConn4 -- PS-Simulink Converter12/LConn1
  joint_4_r/RConn3 -- PS-Simulink Converter15/LConn1
  PS-Simulink Converter14/LConn1 -- joint_4_r/RConn2
  joint_5_b/RConn5 -- PS-Simulink Converter17/LConn1
  joint_5_b/RConn3 -- PS-Simulink Converter19/LConn1
  joint_5_b/RConn2 -- PS-Simulink Converter18/LConn1
  joint_5_b/RConn4 -- PS-Simulink Converter16/LConn1
  joint_6_t/RConn4 -- PS-Simulink Converter32/LConn1
  joint_6_t/RConn2 -- PS-Simulink Converter34/LConn1
  joint_6_t/RConn3 -- PS-Simulink Converter35/LConn1
  joint_6_t/RConn5 -- PS-Simulink Converter33/LConn1
  gripper_finger_joint_l/LConn1 -- gripper_palm_link/RConn2
  gripper_finger_joint_l/RConn1 -- gripper_finger_link_l/LConn1
  gripper_palm_joint/LConn1 -- tool0/RConn1
  gripper_palm_joint/RConn1 -- gripper_palm_link/LConn1
  EE Frame/RConn1 -- gripper_EE_joint/RConn1 -- Transform Sensor/RConn1
  gripper_finger_joint_r/RConn1 -- gripper_finger_link_r/LConn1
  gripper_finger_joint_r/LConn1 -- gripper_palm_link/RConn1
  Simulink-PS Converter1/RConn1 -- gripper_finger_joint_r/LConn2
  Simulink-PS Converter2/RConn1 -- gripper_finger_joint_l/LConn2
  PS-Simulink Converter21/LConn1 -- gripper_finger_joint_r/RConn5
  PS-Simulink Converter23/LConn1 -- gripper_finger_joint_r/RConn3
  PS-Simulink Converter22/LConn1 -- gripper_finger_joint_r/RConn2
  PS-Simulink Converter20/LConn1 -- gripper_finger_joint_r/RConn4
  gripper_finger_joint_l/RConn4 -- PS-Simulink Converter28/LConn1
  gripper_finger_joint_l/RConn2 -- PS-Simulink Converter30/LConn1
  gripper_finger_joint_l/RConn3 -- PS-Simulink Converter31/LConn1
  gripper_finger_joint_l/RConn5 -- PS-Simulink Converter29/LConn1
  world/LConn1 -- world1/RConn1
  world/RConn1 -- base_link1/LConn1

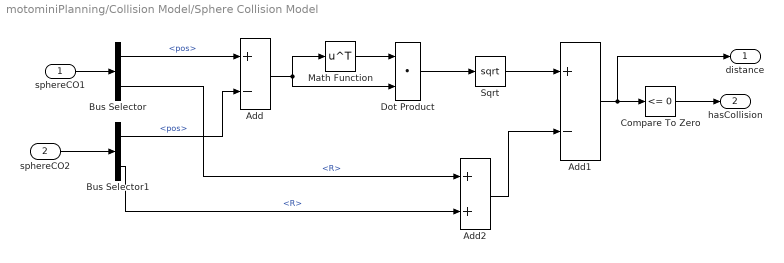
== system motominiPlanning/Collision Model/Sphere Collision Model ==
  sphereCO1 : Inport
  sphereCO2 : Inport  Port=2
  Add : Sum  Inputs=+-
  Add1 : Sum  Inputs=+-
  Add2 : Sum
  Bus Selector : BusSelector  OutputSignals=pos,R
  Bus Selector1 : BusSelector  OutputSignals=pos,R
  Compare To Zero : simulink/Logic and Bit Operations/Compare To Zero  relop=<=  OutDataTypeStr=boolean
  Dot Product : DotProduct  InputSameDT=on  OutDataTypeStr=Inherit: Inherit via internal rule
  Math Function : Math  Operator=transpose  SaturateOnIntegerOverflow=on
  Sqrt : Sqrt  SaturateOnIntegerOverflow=on
  distance : Outport
  hasCollision : Outport  Port=2
  wires:
  sphereCO2/1 -> Bus Selector1/1
  sphereCO1/1 -> Bus Selector/1
  Add2/1 -> Add1/2
  Sqrt/1 -> Add1/1
  Compare To Zero/1 -> hasCollision/1
  Math Function/1 -> Dot Product/1
  Add/1 -> Math Function/1, Dot Product/2
  Dot Product/1 -> Sqrt/1
  Add1/1 -> distance/1, Compare To Zero/1
  Bus Selector/1 -> Add/1  "<pos>"
  Bus Selector1/1 -> Add/2  "<pos>"
  Bus Selector/2 -> Add2/1  "<R>"
  Bus Selector1/2 -> Add2/2  "<R>"

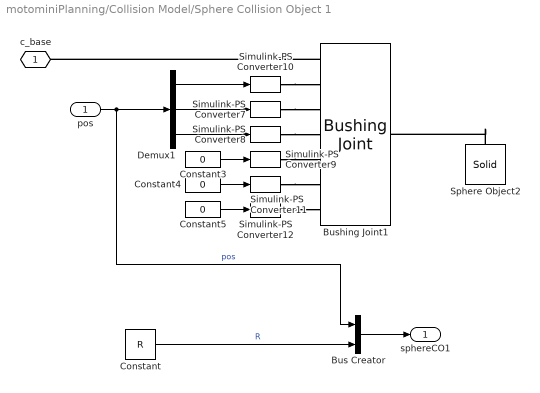
== system motominiPlanning/Collision Model/Sphere Collision Object 1 ==
  pos : Inport
  Bus Creator : BusCreator  Inputs=2
  Bushing Joint1 : sm_lib/Joints/Bushing Joint  SenseConstraintForce=off  SenseConstraintForceX=off  SenseConstraintForceY=off  SenseConstraintForceZ=off  SenseConstraintTorque=off  SenseConstraintTorqueX=off  SenseConstraintTorqueY=off  SenseConstraintTorqueZ=off  SenseTotalForce=off  SenseTotalForceX=off  SenseTotalForceY=off  SenseTotalForceZ=off  SenseTotalTorque=off  SenseTotalTorqueX=off  SenseTotalTorqueY=off  SenseTotalTorqueZ=off  CompositeWrenchDir=FollowerOnBase  CompositeWrenchFrame=BaseFrame  PxEquilibriumPosition=0  PxEquilibriumPositionUnits=m  PxSpringStiffness=0  PxSpringStiffnessUnits=N/m  PxDampingCoefficient=0  PxDampingCoefficientUnits=N/(m/s)  PxTorqueActuationMode=ComputedTorque  PxMotionActuationMode=InputMotion  PxSensePosition=off  PxSenseVelocity=off  PxSenseAcceleration=off  PxSenseTorqueForce=off  PxSenseLowerLimitTorqueForce=off  PxSenseUpperLimitTorqueForce=off  PxLowerLimitSpecify=off  PxLowerLimitBound=-1  PxLowerLimitBoundUnits=m  PxLowerLimitStiffness=1e6  PxLowerLimitStiffnessUnits=N/m  PxLowerLimitDamping=1e3  PxLowerLimitDampingUnits=N/(m/s)  PxLowerLimitTransitionRegionWidth=1e-4  PxLowerLimitTransitionRegionWidthUnits=m  PxUpperLimitSpecify=off  PxUpperLimitBound=1  PxUpperLimitBoundUnits=m  PxUpperLimitStiffness=1e6  PxUpperLimitStiffnessUnits=N/m  PxUpperLimitDamping=1e3  PxUpperLimitDampingUnits=N/(m/s)  PxUpperLimitTransitionRegionWidth=1e-4  PxUpperLimitTransitionRegionWidthUnits=m  PxPositionTargetSpecify=off  PxPositionTargetPriority=High  PxPositionTargetValue=0  PxPositionTargetValueUnits=m  PxVelocityTargetSpecify=off  PxVelocityTargetPriority=High  PxVelocityTargetValue=0  PxVelocityTargetValueUnits=m/s  PyEquilibriumPosition=0  PyEquilibriumPositionUnits=m  PySpringStiffness=0  PySpringStiffnessUnits=N/m  PyDampingCoefficient=0  PyDampingCoefficientUnits=N/(m/s)  PyTorqueActuationMode=ComputedTorque  PyMotionActuationMode=InputMotion  PySensePosition=off  PySenseVelocity=off  PySenseAcceleration=off  PySenseTorqueForce=off  PySenseLowerLimitTorqueForce=off  PySenseUpperLimitTorqueForce=off  PyLowerLimitSpecify=off  PyLowerLimitBound=-1  PyLowerLimitBoundUnits=m  PyLowerLimitStiffness=1e6  PyLowerLimitStiffnessUnits=N/m  PyLowerLimitDamping=1e3  PyLowerLimitDampingUnits=N/(m/s)  PyLowerLimitTransitionRegionWidth=1e-4  PyLowerLimitTransitionRegionWidthUnits=m  PyUpperLimitSpecify=off  PyUpperLimitBound=1  PyUpperLimitBoundUnits=m  PyUpperLimitStiffness=1e6  PyUpperLimitStiffnessUnits=N/m  PyUpperLimitDamping=1e3  PyUpperLimitDampingUnits=N/(m/s)  PyUpperLimitTransitionRegionWidth=1e-4  PyUpperLimitTransitionRegionWidthUnits=m  PyPositionTargetSpecify=off  PyPositionTargetPriority=High  PyPositionTargetValue=0  PyPositionTargetValueUnits=m  PyVelocityTargetSpecify=off  PyVelocityTargetPriority=High  PyVelocityTargetValue=0  PyVelocityTargetValueUnits=m/s  PzEquilibriumPosition=0  PzEquilibriumPositionUnits=m  PzSpringStiffness=0  PzSpringStiffnessUnits=N/m  PzDampingCoefficient=0  PzDampingCoefficientUnits=N/(m/s)  PzTorqueActuationMode=ComputedTorque  PzMotionActuationMode=InputMotion  PzSensePosition=off  PzSenseVelocity=off  PzSenseAcceleration=off  PzSenseTorqueForce=off  PzSenseLowerLimitTorqueForce=off  PzSenseUpperLimitTorqueForce=off  PzLowerLimitSpecify=off  PzLowerLimitBound=-1  PzLowerLimitBoundUnits=m  PzLowerLimitStiffness=1e6  PzLowerLimitStiffnessUnits=N/m  PzLowerLimitDamping=1e3  PzLowerLimitDampingUnits=N/(m/s)  PzLowerLimitTransitionRegionWidth=1e-4  PzLowerLimitTransitionRegionWidthUnits=m  PzUpperLimitSpecify=off  PzUpperLimitBound=1  PzUpperLimitBoundUnits=m  PzUpperLimitStiffness=1e6  PzUpperLimitStiffnessUnits=N/m  PzUpperLimitDamping=1e3  PzUpperLimitDampingUnits=N/(m/s)  PzUpperLimitTransitionRegionWidth=1e-4  PzUpperLimitTransitionRegionWidthUnits=m  PzPositionTargetSpecify=off  PzPositionTargetPriority=High  PzPositionTargetValue=0  PzPositionTargetValueUnits=m  PzVelocityTargetSpecify=off  PzVelocityTargetPriority=High  PzVelocityTargetValue=0  PzVelocityTargetValueUnits=m/s  RxEquilibriumPosition=0  RxEquilibriumPositionUnits=deg  RxSpringStiffness=0  RxSpringStiffnessUnits=N*m/deg  RxDampingCoefficient=0  RxDampingCoefficientUnits=N*m/(deg/s)  RxTorqueActuationMode=ComputedTorque  RxMotionActuationMode=InputMotion  RxSensePosition=off  RxSenseVelocity=off  RxSenseAcceleration=off  RxSenseTorqueForce=off  RxSenseLowerLimitTorqueForce=off  RxSenseUpperLimitTorqueForce=off  RxLowerLimitSpecify=off  RxLowerLimitBound=-90  RxLowerLimitBoundUnits=deg  RxLowerLimitStiffness=1e4  RxLowerLimitStiffnessUnits=N*m/deg  RxLowerLimitDamping=10  RxLowerLimitDampingUnits=N*m/(deg/s)  RxLowerLimitTransitionRegionWidth=0.1  RxLowerLimitTransitionRegionWidthUnits=deg  RxUpperLimitSpecify=off  RxUpperLimitBound=90  RxUpperLimitBoundUnits=deg  RxUpperLimitStiffness=1e4  RxUpperLimitStiffnessUnits=N*m/deg  RxUpperLimitDamping=10  RxUpperLimitDampingUnits=N*m/(deg/s)  RxUpperLimitTransitionRegionWidth=0.1  RxUpperLimitTransitionRegionWidthUnits=deg  RxPositionTargetSpecify=off  RxPositionTargetPriority=High  RxPositionTargetValue=0  RxPositionTargetValueUnits=deg  RxVelocityTargetSpecify=off  RxVelocityTargetPriority=High  RxVelocityTargetValue=0  RxVelocityTargetValueUnits=deg/s  RyEquilibriumPosition=0  RyEquilibriumPositionUnits=deg  RySpringStiffness=0  RySpringStiffnessUnits=N*m/deg  RyDampingCoefficient=0  RyDampingCoefficientUnits=N*m/(deg/s)  RyTorqueActuationMode=ComputedTorque  RyMotionActuationMode=InputMotion  RySensePosition=off  RySenseVelocity=off  RySenseAcceleration=off  RySenseTorqueForce=off  RySenseLowerLimitTorqueForce=off  RySenseUpperLimitTorqueForce=off  RyLowerLimitSpecify=off  RyLowerLimitBound=-90  RyLowerLimitBoundUnits=deg  RyLowerLimitStiffness=1e4  RyLowerLimitStiffnessUnits=N*m/deg  RyLowerLimitDamping=10  RyLowerLimitDampingUnits=N*m/(deg/s)  RyLowerLimitTransitionRegionWidth=0.1  RyLowerLimitTransitionRegionWidthUnits=deg  RyUpperLimitSpecify=off  RyUpperLimitBound=90  RyUpperLimitBoundUnits=deg  RyUpperLimitStiffness=1e4  RyUpperLimitStiffnessUnits=N*m/deg  RyUpperLimitDamping=10  RyUpperLimitDampingUnits=N*m/(deg/s)  RyUpperLimitTransitionRegionWidth=0.1  RyUpperLimitTransitionRegionWidthUnits=deg  RyPositionTargetSpecify=off  RyPositionTargetPriority=High  RyPositionTargetValue=0  RyPositionTargetValueUnits=deg  RyVelocityTargetSpecify=off  RyVelocityTargetPriority=High  RyVelocityTargetValue=0  RyVelocityTargetValueUnits=deg/s  RzEquilibriumPosition=0  RzEquilibriumPositionUnits=deg  RzSpringStiffness=0  RzSpringStiffnessUnits=N*m/deg  RzDampingCoefficient=0  RzDampingCoefficientUnits=N*m/(deg/s)  RzTorqueActuationMode=ComputedTorque  RzMotionActuationMode=InputMotion  RzSensePosition=off  RzSenseVelocity=off  RzSenseAcceleration=off  RzSenseTorqueForce=off  RzSenseLowerLimitTorqueForce=off  RzSenseUpperLimitTorqueForce=off  RzLowerLimitSpecify=off  RzLowerLimitBound=-90  RzLowerLimitBoundUnits=deg  RzLowerLimitStiffness=1e4  RzLowerLimitStiffnessUnits=N*m/deg  RzLowerLimitDamping=10  RzLowerLimitDampingUnits=N*m/(deg/s)  RzLowerLimitTransitionRegionWidth=0.1  RzLowerLimitTransitionRegionWidthUnits=deg  RzUpperLimitSpecify=off  RzUpperLimitBound=90  RzUpperLimitBoundUnits=deg  RzUpperLimitStiffness=1e4  RzUpperLimitStiffnessUnits=N*m/deg  RzUpperLimitDamping=10  RzUpperLimitDampingUnits=N*m/(deg/s)  RzUpperLimitTransitionRegionWidth=0.1  RzUpperLimitTransitionRegionWidthUnits=deg  RzPositionTargetSpecify=off  RzPositionTargetPriority=High  RzPositionTargetValue=0  RzPositionTargetValueUnits=deg  RzVelocityTargetSpecify=off  RzVelocityTargetPriority=High  RzVelocityTargetValue=0  RzVelocityTargetValueUnits=deg/s
      settings: SourceProductName=Simscape Multibody
  Constant : Constant  Value=R
  Constant3 : Constant  Value=0
  Constant4 : Constant  Value=0
  Constant5 : Constant  Value=0
  Demux1 : Demux  Outputs=3
  Simulink-PS Converter{7..12} (6 alike) : nesl_utility/Simulink-PS Converter  PhysicalDomain=network_engine_domain  SubClassName=ps_input  LeftPortType=input  RightPortType=output  PseudoPeriodic=off  Frequencies=[]  NoiseDistribution=none  NoiseParameters=[]  Unit=1  AffineConversion=off  FilteringAndDerivatives=filter  SimscapeFilterOrder=2  InputFilterTimeConstant=0.001  UdotUserProvided=1
  Sphere Object2 : sm_lib/Body Elements/Solid  InertiaType=CalculateFromGeometry  Mass=1  MassUnits=kg  CenterOfMass=[0 0 0]  CenterOfMassUnits=m  MomentsOfInertia=[1 1 1]  MomentsOfInertiaUnits=kg*m^2  ProductsOfInertia=[1 1 1]  ProductsOfInertiaUnits=kg*m^2  BasedOnType=Density  Density=1e-3  DensityUnits=kg/m^3  DoExposeReferenceFrame=on  SerializedFrames=<Frames/>  GraphicType=FromGeometry  MarkerShape=Sphere  MarkerSize=10  GraphicVisPropType=SimpleVisualProperties  GraphicDiffuseColor=[1.0 0.2 0.2]  GraphicSpecularColor=[0.5 0.5 0.5 1.0]  GraphicAmbientColor=[0.15 0.15 0.15 1.0]  GraphicEmissiveColor=[0.0 0.0 0.0 1.0]  GraphicShininess=75  GraphicOpacity=0.7  GeometryShape=Sphere  RectangleSize=[1 1]  RectangleSizeUnits=m  BrickDimensions=[1 1 1]  BrickDimensionUnits=m  CylinderRadius=1  CylinderRadiusUnits=m  CylinderLength=1  CylinderLengthUnits=m  SphereRadius=R  SphereRadiusUnits=m  EllipsoidRadii=[1 1 1]  EllipsoidRadiiUnits=m  ExtrusionCrossSection=[1 1; -1 1; -1 -1; 1 -1]  ExtrusionCrossSectionUnits=m  ExtrusionLength=1  ExtrusionLengthUnits=m  PolygonNumSides=3  PolygonOuterRadius=1  PolygonOuterRadiusUnits=m  ExtGeomFileType=STEP  ExtGeomFileUnits=m  RevolutionCrossSection=[1 1; 1 -1; 2 -1; 2 1]  RevolutionCrossSectionUnits=m  RevolutionExtent=Full  RevolutionAngle=180  RevolutionAngleUnits=deg
  c_base : PMIOPort  Side=Left
  sphereCO1 : Outport
  wires:
  Demux1/3 -> Simulink-PS Converter8/1
  Constant4/1 -> Simulink-PS Converter11/1
  Demux1/2 -> Simulink-PS Converter7/1
  Demux1/1 -> Simulink-PS Converter10/1
  pos/1 -> Bus Creator/1, Demux1/1  "pos"
  Constant3/1 -> Simulink-PS Converter9/1
  Constant5/1 -> Simulink-PS Converter12/1
  Constant/1 -> Bus Creator/2  "R"
  Bus Creator/1 -> sphereCO1/1
  connections:
  Bushing Joint1/LConn1 -- c_base/RConn1
  Simulink-PS Converter9/RConn1 -- Bushing Joint1/LConn5
  Simulink-PS Converter10/RConn1 -- Bushing Joint1/LConn2
  Simulink-PS Converter11/RConn1 -- Bushing Joint1/LConn6
  Sphere Object2/RConn1 -- Bushing Joint1/RConn1
  Simulink-PS Converter7/RConn1 -- Bushing Joint1/LConn3
  Simulink-PS Converter12/RConn1 -- Bushing Joint1/LConn7
  Simulink-PS Converter8/RConn1 -- Bushing Joint1/LConn4
